simulink model "DeltaS"  (R2016b)
settings: Solver=VariableStepAuto  StartTime=0.0  StopTime=0.08  RelTol=1e-3
libraries: powerlib x23
settings Model: Creator=Youssef  LastModifiedBy=Youssef

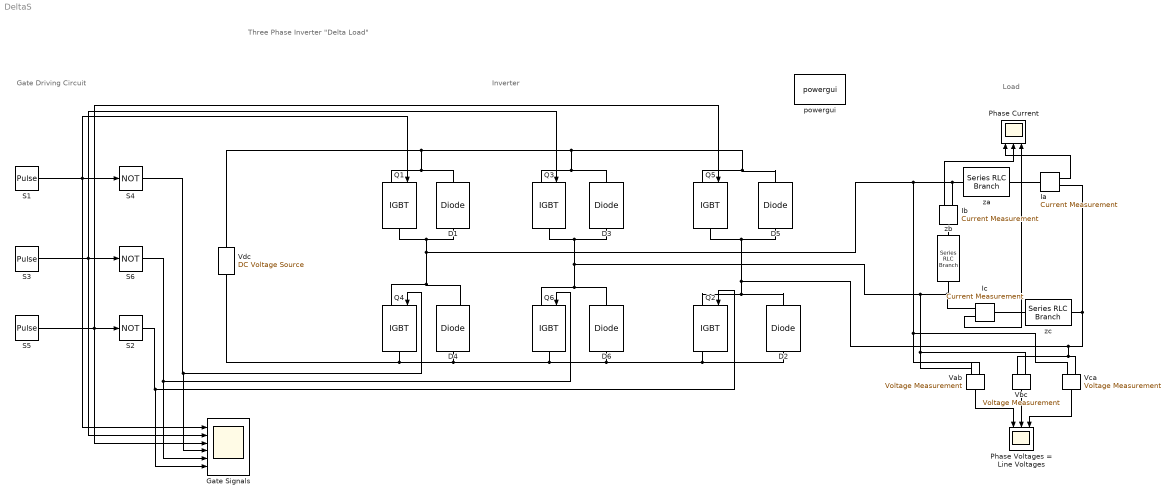
== system DeltaS ==
  note: Gate Driving Circuit
  note: Load
  note: Three Phase Inverter "Delta Load"
  note: Inverter
  D{1..3,5..6} (5 alike) : powerlib/Power Electronics/Diode  Ron=0.001  Lon=0  Vf=0.8  IC=0  UseSnubber=off  Rs=500  Cs=250e-9  Measurements=off
  D4 : powerlib/Power Electronics/Diode  Ron=0.001  Lon=0  Vf=0.8  IC=0  UseSnubber=off  Rs=500  Cs=250e-9  Measurements=on
  Gate Signals : Scope  NumInputPorts=6
  Ia : powerlib/Measurements/Current Measurement  PhasorSimulation=off  OutputType=Complex  PSBequivalent=0
  Ib : powerlib/Measurements/Current Measurement  PhasorSimulation=off  OutputType=Complex  PSBequivalent=0
  Ic : powerlib/Measurements/Current Measurement  PhasorSimulation=off  OutputType=Complex  PSBequivalent=0
  Phase Current : Scope  NumInputPorts=3
  Phase Voltages = Line Voltages : Scope  NumInputPorts=3
  Q{1,3..6} (5 alike) : powerlib/Power Electronics/IGBT  Ron=0.001  Lon=0  Vf=0.4  Tf=1e-6  Tt=2e-6  IC=0  Rs=1e5  Cs=inf  Measurements=off
  Q2 : powerlib/Power Electronics/IGBT  Ron=0.001  Lon=0  Vf=0.4  Tf=1e-6  Tt=2e-6  IC=0  Rs=1e5  Cs=inf  Measurements=on
  S1 : DiscretePulseGenerator  PulseType=Time based  Period=0.02  PulseWidth=50
  S2 : Logic  Operator=NOT  AllPortsSameDT=off  OutDataTypeStr=boolean
  S3 : DiscretePulseGenerator  PulseType=Time based  Period=0.02  PulseWidth=50  PhaseDelay=0.02/3
  S4 : Logic  Operator=NOT  AllPortsSameDT=off  OutDataTypeStr=boolean
  S5 : DiscretePulseGenerator  PulseType=Time based  Period=0.02  PulseWidth=50  PhaseDelay=(2*0.02)/3
  S6 : Logic  Operator=NOT  AllPortsSameDT=off  OutDataTypeStr=boolean
  Vab : powerlib/Measurements/Voltage Measurement  PhasorSimulation=off  OutputType=Complex  PSBequivalent=0
  Vbc : powerlib/Measurements/Voltage Measurement  PhasorSimulation=off  OutputType=Complex  PSBequivalent=0
  Vca : powerlib/Measurements/Voltage Measurement  PhasorSimulation=off  OutputType=Complex  PSBequivalent=0
  Vdc : powerlib/Electrical Sources/DC Voltage Source  Amplitude=282  Measurements=None
  powergui : powerlib/powergui  Priority=1  SimulationMode=Discrete  SolverType=Tustin/Backward Euler (TBE)  SampleTime=1e-6  frequency=60  SPID=off  DisableSnubberDevices=off  DisableRonSwitches=off  DisableVfSwitches=off  SwTol=0  DisplayEquations=off  Interpol=off  ExternalGateDelay=off  methode=off  Ts=10  FunctionMessages=off  echomessages=off  HookPort=off  EnableUseOfTLC=off  x0status=blocks  frequencyindice=0  Pbase=100e6  ErrMax=1e-4  Iterations=50  UnitsV=kV  UnitsW=MW  buscounter=0  RestoreLinks=warning  ResistiveCurrentMeasurement=off  Frange=[0:2:500]  Ylog=off  Xlog=on  ShowGrid=off  save=off  variable=ZData  structure=I  ZoomFFT=off  StartTime=0.02  cycles=2  DisplayStyle=1  fundamental=50  FreqAxis=off  MaxFrequency=1000  frequencyindicesteady=1  RmsSteady=1  display=off
  za : powerlib/Elements/Series RLC Branch  LConnTagsString=__new0  RConnTagsString=__new0  BranchType=RL  Resistance=1  Inductance=1e-3  SetiL0=off  InitialCurrent=0  Capacitance=1e-6  Setx0=off  InitialVoltage=0  Measurements=None
  zb : powerlib/Elements/Series RLC Branch  LConnTagsString=__new0  RConnTagsString=__new0  BranchType=RL  Resistance=1  Inductance=1e-3  SetiL0=off  InitialCurrent=0  Capacitance=1e-6  Setx0=off  InitialVoltage=0  Measurements=None
  zc : powerlib/Elements/Series RLC Branch  LConnTagsString=__new0  RConnTagsString=__new0  BranchType=RL  Resistance=1  Inductance=1e-3  SetiL0=off  InitialCurrent=0  Capacitance=1e-6  Setx0=off  InitialVoltage=0  Measurements=None
  wires:
  S1/1 -> Gate Signals/1, Q1/1, S4/1
  S3/1 -> Gate Signals/2, Q3/1, S6/1
  S5/1 -> Gate Signals/3, Q5/1, S2/1
  S6/1 -> Gate Signals/5, Q6/1
  S4/1 -> Gate Signals/4, Q4/1
  S2/1 -> Gate Signals/6, Q2/1
  Ia/1 -> Phase Current/1
  Ib/1 -> Phase Current/2
  Ic/1 -> Phase Current/3
  Vab/1 -> Phase Voltages = Line Voltages/1
  Vbc/1 -> Phase Voltages = Line Voltages/2
  Vca/1 -> Phase Voltages = Line Voltages/3
  connections:
  Q1/LConn1 -- D1/RConn1 -- Vdc/RConn1 -- D5/RConn1 -- Q5/LConn1 -- Q3/LConn1 -- D3/RConn1
  Q4/RConn1 -- D4/LConn1 -- D2/LConn1 -- Q2/RConn1 -- D6/LConn1 -- Q6/RConn1 -- Vdc/LConn1
  Q1/RConn1 -- D1/LConn1 -- Q4/LConn1 -- D4/RConn1 -- Vca/LConn2 -- Vab/LConn1 -- Ib/RConn1 -- za/LConn1
  D6/RConn1 -- Q6/LConn1 -- Vbc/LConn1 -- Vab/LConn2 -- Ic/RConn1 -- zb/RConn1 -- Q3/RConn1 -- D3/LConn1
  Ia/LConn1 -- za/RConn1
  D5/LConn1 -- Vca/LConn1 -- Vbc/LConn2 -- Ia/RConn1 -- zc/RConn1 -- D2/RConn1 -- Q2/LConn1 -- Q5/RConn1
  Ic/LConn1 -- zc/LConn1
  Ib/LConn1 -- zb/LConn1
